simulink model "RLTunningTV"  (R2019b)
settings: Solver=odeN  StartTime=0.0  StopTime=15  FixedStep=0.001  RelTol=1e-3
PreLoadFcn:
  | Vehicle_parameters;
  | hcc_init;
InitFcn:
  | Vehicle_parameters;
  | hcc_init;
values from neighbouring files (symbols this model uses):
  c = (1.596+1.610)/2    (= 1.603)    [Vehicle_parameters.m]
  g = 9.8    [Vehicle_parameters.m]
  gamma = 0.006    [hcc_init.m]
  Jzz = 2050    [Vehicle_parameters.m]
  kx1 = 0.05890269    [hcc_init.m]
  ky1 = 0.04086363    [hcc_init.m]
  kz1 = 0.27516026    [hcc_init.m]
  lf = 1.3265    [Vehicle_parameters.m]
  lr = 1.3685    [Vehicle_parameters.m]
  M = 1360    [Vehicle_parameters.m]
  n = 6    [hcc_init.m]    (also in smoothing_t0.m = 16)
  pbk_gain = 1.0    (= 1)    [hcc_init.m]
  Q_gain = 50.0    (= 50)    [hcc_init.m]
  Qf = [0.0, 0.0 ... (first row only)    [hcc_init.m]
  Qr = [0.0, 0.0 ... (first row only)    [hcc_init.m]
  Reff = 0.323    [Vehicle_parameters.m]
  swa_gain = 45.0    (= 45)    [hcc_init.m]
  umax_m = 4000.0    (= 4000)    [hcc_init.m]
  umin_br = umin_m + umin_b    (= -4500)    [hcc_init.m]
  v = 80    [Vehicle_parameters.m]
  wFx = 0.4    [hcc_init.m]
  wFy = 0.02    [hcc_init.m]
  wGz = 1500.89459504    [hcc_init.m]
undefined symbols (not defined in the file or in its folder): DiscIntNeverNeededParam, LMUX, LMUY, sigbuilder_block
libraries: simulink x10, rllib x1
(part 2 of 3)

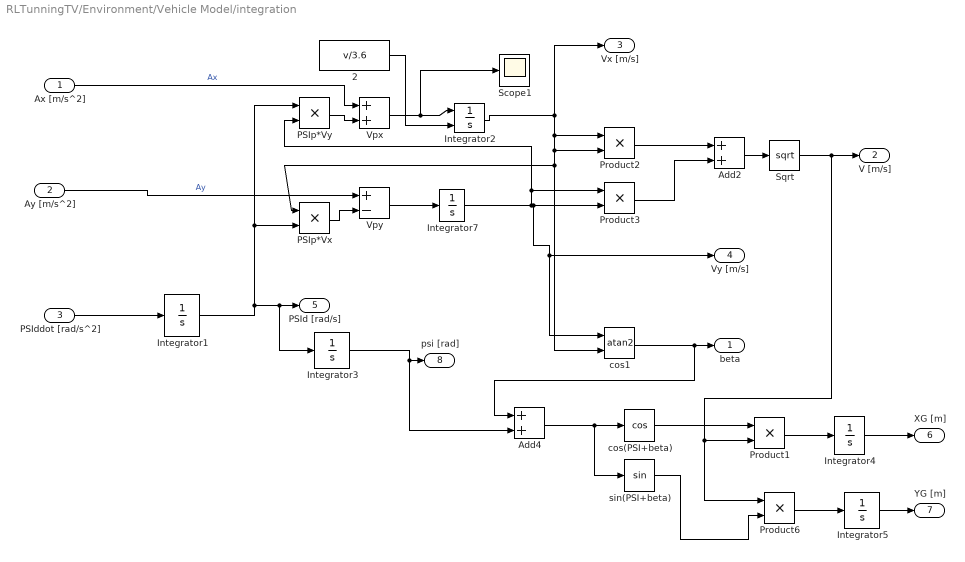
== system RLTunningTV/Environment/Vehicle Model/integration ==
  Ax [m/s^2] : Inport
  Ay [m/s^2] : Inport  Port=2
  PSIddot [rad/s^2] : Inport  Port=3
  2 : Constant  Value=v/3.6
  Add2 : Sum
  Add4 : Sum
  Integrator{1,3..5,7} (5 alike) : Integrator
  Integrator2 : Integrator  InitialConditionSource=external  InitialCondition=v/3.6
  PSIp*Vx : Product  RndMeth=Zero
  PSIp*Vy : Product  RndMeth=Zero
  Product{1..3,6} (4 alike) : Product  RndMeth=Zero
  Scope1 : Scope
  Sqrt : Sqrt  SaturateOnIntegerOverflow=on
  Vpx : Sum
  Vpy : Sum  Inputs=+-
  cos(PSI+beta) : Trigonometry  Operator=cos
  cos1 : Trigonometry  Operator=atan2
  sin(PSI+beta) : Trigonometry
  beta : Outport  VectorParamsAs1DForOutWhenUnconnected=off
  V [m/s] : Outport  Port=2  VectorParamsAs1DForOutWhenUnconnected=off
  Vx [m/s] : Outport  Port=3  VectorParamsAs1DForOutWhenUnconnected=off
  Vy [m/s] : Outport  Port=4  VectorParamsAs1DForOutWhenUnconnected=off
  PSId [rad/s] : Outport  Port=5  VectorParamsAs1DForOutWhenUnconnected=off
  XG [m] : Outport  Port=6  VectorParamsAs1DForOutWhenUnconnected=off
  YG [m] : Outport  Port=7  VectorParamsAs1DForOutWhenUnconnected=off
  psi [rad] : Outport  Port=8  VectorParamsAs1DForOutWhenUnconnected=off
  wires:
  Vpx/1 -> Integrator2/1, Scope1/1
  Integrator5/1 -> YG [m]/1
  Integrator4/1 -> XG [m]/1
  Product1/1 -> Integrator4/1
  Product6/1 -> Integrator5/1
  Add4/1 -> sin(PSI+beta)/1, cos(PSI+beta)/1
  sin(PSI+beta)/1 -> Product6/2
  cos(PSI+beta)/1 -> Product1/1
  Integrator3/1 -> psi [rad]/1, Add4/2
  Sqrt/1 -> Product6/1, Product1/2, V [m/s]/1
  Add2/1 -> Sqrt/1
  Product3/1 -> Add2/2
  Product2/1 -> Add2/1
  cos1/1 -> Add4/1, beta/1
  Ay [m/s^2]/1 -> Vpy/1  "Ay"
  Integrator7/1 -> Product3/2, cos1/1, Vy [m/s]/1, PSIp*Vy/2, Product3/1
  Vpy/1 -> Integrator7/1
  PSIp*Vx/1 -> Vpy/2
  PSIp*Vy/1 -> Vpx/2
  Ax [m/s^2]/1 -> Vpx/1  "Ax"
  Integrator2/1 -> Vx [m/s]/1, PSIp*Vx/1, cos1/2, Product2/2, Product2/1
  PSIddot [rad/s^2]/1 -> Integrator1/1
  Integrator1/1 -> PSIp*Vx/2, PSIp*Vy/1, PSId [rad/s]/1, Integrator3/1
  2/1 -> Integrator2/2

== system RLTunningTV/Environment/Vehicle Model/lateral slip ==
  steering : Inport
  vx : Inport  Port=2
  vy : Inport  Port=3
  psid : Inport  Port=4
  Mux : Mux
  Scope : Scope
  alpha_FL : Subsystem  TreatAsAtomicUnit=on
  alpha_FR : Subsystem  TreatAsAtomicUnit=on
  alpha_RL : Subsystem  TreatAsAtomicUnit=on
  alpha_RR : Subsystem  TreatAsAtomicUnit=on
  alpha[4x1] : Outport  VectorParamsAs1DForOutWhenUnconnected=off
  wires:
  alpha_RL/1(alpha_RL) -> Mux/4
  alpha_RR/1(alpha_RR) -> Mux/3
  alpha_FL/1(alpha_FL) -> Mux/2
  alpha_FR/1(alpha_FR) -> Mux/1, Scope/1
  Mux/1 -> alpha[4x1]/1
  psid/1 -> alpha_FR/4(psid), alpha_FL/4(psid), alpha_RR/3(psid), alpha_RL/3(psid)
  vy/1 -> alpha_FR/3(vy), alpha_FL/3(vy), alpha_RR/2(vy), alpha_RL/2(vy)
  vx/1 -> alpha_FR/2(vx), alpha_FL/2(vx), alpha_RR/1(vx), alpha_RL/1(vx)
  steering/1 -> alpha_FR/1(steering), alpha_FL/1(steering)

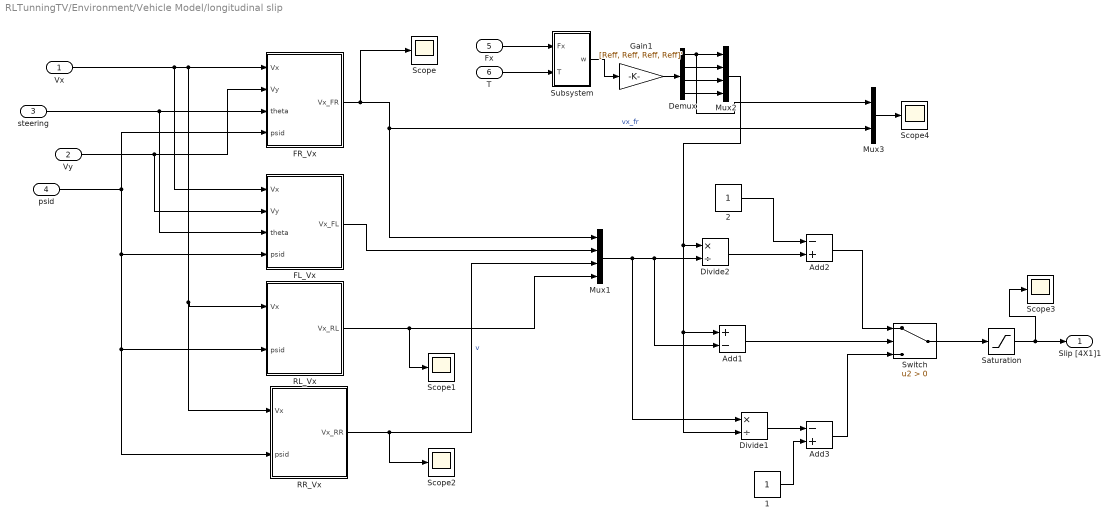
== system RLTunningTV/Environment/Vehicle Model/longitudinal slip ==
  Vx : Inport
  Vy : Inport  Port=2
  steering : Inport  Port=3
  psid : Inport  Port=4
  Fx : Inport  Port=5
  T : Inport  Port=6
  1 : Constant
  2 : Constant
  Add1 : Sum  Inputs=+-
  Add2 : Sum  Inputs=-+
  Add3 : Sum  Inputs=-+
  Demux : Demux
  Divide1 : Product  Inputs=*/
  Divide2 : Product  Inputs=*/
  FL_Vx : Subsystem  TreatAsAtomicUnit=on
  FR_Vx : Subsystem  TreatAsAtomicUnit=on
  Gain1 : Gain  Gain=[Reff, Reff, Reff, Reff]'
  Mux1 : Mux
  Mux2 : Mux
  Mux3 : Mux  Inputs=2
  RL_Vx : Subsystem  TreatAsAtomicUnit=on
  RR_Vx : Subsystem  TreatAsAtomicUnit=on
  Saturation : Saturate  UpperLimit=1  LowerLimit=-1
  Scope{,1..4} (5 alike) : Scope
  Subsystem : Subsystem
  Switch : Switch  Criteria=u2 > Threshold
  Slip [4X1]1 : Outport  VectorParamsAs1DForOutWhenUnconnected=off
  wires:
  T/1 -> Subsystem/2(T)
  Fx/1 -> Subsystem/1(Fx)
  Gain1/1 -> Demux/1
  Add2/1 -> Switch/1
  Add3/1 -> Switch/3
  1/1 -> Add3/2
  Divide1/1 -> Add3/1
  Add1/1 -> Switch/2
  Mux1/1 -> Divide2/2, Add1/2, Divide1/1
  RL_Vx/1(Vx_RL) -> Mux1/4, Scope1/1
  RR_Vx/1(Vx_RR) -> Mux1/3, Scope2/1  "v"
  FL_Vx/1(Vx_FL) -> Mux1/2
  FR_Vx/1(Vx_FR) -> Mux3/2, Mux1/1, Scope/1  "vx_fr"
  2/1 -> Add2/1
  Divide2/1 -> Add2/2
  steering/1 -> FR_Vx/3(theta), FL_Vx/3(theta)
  Vy/1 -> FR_Vx/2(Vy), FL_Vx/2(Vy)
  Subsystem/1(w) -> Gain1/1
  psid/1 -> FR_Vx/4(psid), RL_Vx/2(psid), RR_Vx/2(psid), FL_Vx/4(psid)
  Vx/1 -> RL_Vx/1(Vx), RR_Vx/1(Vx), FR_Vx/1(Vx), FL_Vx/1(Vx)
  Saturation/1 -> Scope3/1, Slip [4X1]1/1
  Demux/1 -> Mux3/1, Mux2/1
  Demux/2 -> Mux2/2
  Demux/3 -> Mux2/3
  Demux/4 -> Mux2/4
  Mux2/1 -> Divide1/2, Add1/1, Divide2/1
  Mux3/1 -> Scope4/1
  Switch/1 -> Saturation/1

== system RLTunningTV/Environment/DCIM/lateral slip/alpha_FL ==
  steering : Inport
  vx : Inport  Port=2
  vy : Inport  Port=3
  psid : Inport  Port=4
  Add : Sum  Inputs=+-
  Add1 : Sum  Inputs=-+
  Add2 : Sum
  Add3 : Sum
  Divide : Product  Inputs=*/
  Gain1 : Gain  Gain=lf
  Product{,1..3} (4 alike) : Product  RndMeth=Zero
  Trigonometric Function2 : Trigonometry  Operator=atan
  cos theta : Trigonometry  Operator=cos
  psid*c : Gain  Gain=c
  sin theta : Trigonometry
  alpha_FL : Outport  VectorParamsAs1DForOutWhenUnconnected=off
  wires:
  vx/1 -> Add/1
  psid/1 -> Gain1/1, psid*c/1
  psid*c/1 -> Add/2
  Add/1 -> Product1/1, Product/1
  steering/1 -> sin theta/1, cos theta/1
  sin theta/1 -> Product2/1, Product/2
  cos theta/1 -> Product3/1, Product1/2
  Product/1 -> Add1/1
  Product1/1 -> Add2/1
  Gain1/1 -> Add3/1
  vy/1 -> Add3/2
  Add3/1 -> Product2/2, Product3/2
  Product2/1 -> Add2/2
  Product3/1 -> Add1/2
  Add1/1 -> Divide/1
  Add2/1 -> Divide/2
  Divide/1 -> Trigonometric Function2/1
  Trigonometric Function2/1 -> alpha_FL/1

== system RLTunningTV/Environment/DCIM/lateral slip/alpha_FR ==
  steering : Inport
  vx : Inport  Port=2
  vy : Inport  Port=3
  psid : Inport  Port=4
  Add : Sum
  Add1 : Sum  Inputs=-+
  Add2 : Sum
  Add3 : Sum
  Divide : Product  Inputs=*/
  Gain : Gain  Gain=c
  Gain1 : Gain  Gain=lf
  Product{,1..3} (4 alike) : Product  RndMeth=Zero
  Trigonometric Function : Trigonometry
  Trigonometric Function1 : Trigonometry  Operator=cos
  Trigonometric Function2 : Trigonometry  Operator=atan
  alpha_FR : Outport  VectorParamsAs1DForOutWhenUnconnected=off
  wires:
  vx/1 -> Add/1
  psid/1 -> Gain1/1, Gain/1
  Gain/1 -> Add/2
  Add/1 -> Product1/1, Product/1
  steering/1 -> Trigonometric Function/1, Trigonometric Function1/1
  Trigonometric Function/1 -> Product2/1, Product/2
  Trigonometric Function1/1 -> Product3/1, Product1/2
  Product/1 -> Add1/1
  Product1/1 -> Add2/1
  Gain1/1 -> Add3/1
  vy/1 -> Add3/2
  Add3/1 -> Product2/2, Product3/2
  Product2/1 -> Add2/2
  Product3/1 -> Add1/2
  Add1/1 -> Divide/1
  Add2/1 -> Divide/2
  Divide/1 -> Trigonometric Function2/1
  Trigonometric Function2/1 -> alpha_FR/1

== system RLTunningTV/Environment/DCIM/lateral slip/alpha_RL ==
  vx : Inport
  vy : Inport  Port=2
  psid : Inport  Port=3
  Add : Sum  Inputs=+-
  Add3 : Sum  Inputs=-+
  Divide : Product  Inputs=*/
  Gain : Gain  Gain=c
  Gain1 : Gain  Gain=lr
  Trigonometric Function2 : Trigonometry  Operator=atan
  alpha_RL : Outport  VectorParamsAs1DForOutWhenUnconnected=off
  wires:
  vx/1 -> Add/1
  psid/1 -> Gain1/1, Gain/1
  Gain/1 -> Add/2
  Add/1 -> Divide/2
  Gain1/1 -> Add3/1
  vy/1 -> Add3/2
  Add3/1 -> Divide/1
  Divide/1 -> Trigonometric Function2/1
  Trigonometric Function2/1 -> alpha_RL/1

== system RLTunningTV/Environment/DCIM/lateral slip/alpha_RR ==
  vx : Inport
  vy : Inport  Port=2
  psid : Inport  Port=3
  Add : Sum
  Add3 : Sum  Inputs=-+
  Divide : Product  Inputs=*/
  Gain : Gain  Gain=c
  Gain1 : Gain  Gain=lr
  Trigonometric Function2 : Trigonometry  Operator=atan
  alpha_RR : Outport  VectorParamsAs1DForOutWhenUnconnected=off
  wires:
  vx/1 -> Add/1
  psid/1 -> Gain1/1, Gain/1
  Gain/1 -> Add/2
  Add/1 -> Divide/2
  Gain1/1 -> Add3/1
  vy/1 -> Add3/2
  Add3/1 -> Divide/1
  Divide/1 -> Trigonometric Function2/1
  Trigonometric Function2/1 -> alpha_RR/1

== system RLTunningTV/Environment/DCIM/longitudinal slip/FL_Vx ==
  Vx : Inport
  Vy : Inport  Port=2
  theta : Inport  Port=3
  psid : Inport  Port=4
  (Vx+PSIp*lf)*sin(theta) : Product  RndMeth=Zero
  (Vx+PSIp*lf)*sin(theta)1 : Product  RndMeth=Zero
  Vx+PSId*lf : Sum
  Vx+PSId*lf1 : Sum  Inputs=+-
  Vx1 : Sum
  cos delta : Trigonometry  Operator=cos
  psip ca/1 : Gain  Gain=c
  psip ca/2 : Gain  Gain=lf
  sin delta : Trigonometry
  Vx_FL : Outport  VectorParamsAs1DForOutWhenUnconnected=off
  wires:
  Vy/1 -> Vx+PSId*lf/1
  psid/1 -> psip ca/1/1, psip ca/2/1
  psip ca/2/1 -> Vx+PSId*lf/2
  Vx+PSId*lf/1 -> (Vx+PSIp*lf)*sin(theta)/1
  theta/1 -> cos delta/1, sin delta/1
  sin delta/1 -> (Vx+PSIp*lf)*sin(theta)/2
  Vx1/1 -> Vx_FL/1
  (Vx+PSIp*lf)*sin(theta)/1 -> Vx1/1
  cos delta/1 -> (Vx+PSIp*lf)*sin(theta)1/1
  Vx/1 -> Vx+PSId*lf1/1
  psip ca/1/1 -> Vx+PSId*lf1/2
  Vx+PSId*lf1/1 -> (Vx+PSIp*lf)*sin(theta)1/2
  (Vx+PSIp*lf)*sin(theta)1/1 -> Vx1/2

== system RLTunningTV/Environment/DCIM/longitudinal slip/FR_Vx ==
  Vx : Inport
  Vy : Inport  Port=2
  theta : Inport  Port=3
  psid : Inport  Port=4
  (Vx+PSIp*lf)*sin(theta)1 : Product  RndMeth=Zero
  (Vy+PSIp*lf)*sin(theta) : Product  RndMeth=Zero
  Vx+PSId*lf : Sum
  Vx+PSId*lf1 : Sum
  Vx2 : Sum
  cos delta : Trigonometry  Operator=cos
  psip ca/1 : Gain  Gain=c
  psip ca/3 : Gain  Gain=lf
  sin delta : Trigonometry
  Vx_FR : Outport  VectorParamsAs1DForOutWhenUnconnected=off
  wires:
  psip ca/3/1 -> Vx+PSId*lf/1
  psid/1 -> psip ca/1/1, psip ca/3/1
  Vx+PSId*lf/1 -> (Vy+PSIp*lf)*sin(theta)/1
  theta/1 -> sin delta/1, cos delta/1
  sin delta/1 -> (Vy+PSIp*lf)*sin(theta)/2
  Vx2/1 -> Vx_FR/1
  (Vy+PSIp*lf)*sin(theta)/1 -> Vx2/1
  cos delta/1 -> (Vx+PSIp*lf)*sin(theta)1/1
  psip ca/1/1 -> Vx+PSId*lf1/2
  Vx+PSId*lf1/1 -> (Vx+PSIp*lf)*sin(theta)1/2
  (Vx+PSIp*lf)*sin(theta)1/1 -> Vx2/2
  Vy/1 -> Vx+PSId*lf/2
  Vx/1 -> Vx+PSId*lf1/1

== system RLTunningTV/Environment/DCIM/longitudinal slip/RL_Vx ==
  Vx : Inport
  psid : Inport  Port=2
  Vx-PSId*c : Sum  Inputs=+-
  psip c : Gain  Gain=c
  Vx_RL : Outport  VectorParamsAs1DForOutWhenUnconnected=off
  wires:
  psid/1 -> psip c/1
  Vx-PSId*c/1 -> Vx_RL/1
  Vx/1 -> Vx-PSId*c/1
  psip c/1 -> Vx-PSId*c/2

== system RLTunningTV/Environment/DCIM/longitudinal slip/RR_Vx ==
  Vx : Inport
  psid : Inport  Port=2
  Vx+PSId*c : Sum
  psip c : Gain  Gain=c
  Vx_RR : Outport  VectorParamsAs1DForOutWhenUnconnected=off
  wires:
  psid/1 -> psip c/1
  Vx+PSId*c/1 -> Vx_RR/1
  Vx/1 -> Vx+PSId*c/1
  psip c/1 -> Vx+PSId*c/2

== system RLTunningTV/Environment/DCIM/longitudinal slip/Subsystem ==
  Fx : Inport
  T : Inport  Port=2
  1/J : Gain  Gain=1./[1.04, 1.04, 1.04 ,1.04]'
  2 : Constant  Value=v/3.6*1/Reff
  Add : Sum  Inputs=-+
  Demux : Demux
  Discrete-Time Integrator{,1..3} (4 alike) : DiscreteIntegrator  InitialConditionSource=external  InitialCondition=v/3.6*1/Reff  SampleTime=0.001  ICPrevOutput=DiscIntNeverNeededParam  ICPrevScaledInput=DiscIntNeverNeededParam
  Mux : Mux
  Reff : Gain  Gain=[Reff, Reff, Reff, Reff]'
  Saturation : Saturate  UpperLimit=inf  LowerLimit=0
  Scope : Scope
  Scope1 : Scope
  w : Outport  VectorParamsAs1DForOutWhenUnconnected=off
  wires:
  Add/1 -> 1/J/1
  Reff/1 -> Add/1
  Saturation/1 -> w/1
  Fx/1 -> Reff/1
  T/1 -> Add/2
  1/J/1 -> Demux/1, Scope/1  "omegap"
  Demux/3 -> Discrete-Time Integrator2/1
  Demux/2 -> Discrete-Time Integrator1/1
  Demux/4 -> Discrete-Time Integrator3/1
  Demux/1 -> Discrete-Time Integrator/1
  Discrete-Time Integrator2/1 -> Mux/3  "omega"
  Discrete-Time Integrator1/1 -> Mux/2
  Discrete-Time Integrator3/1 -> Mux/4
  Discrete-Time Integrator/1 -> Mux/1
  Mux/1 -> Saturation/1, Scope1/1
  2/1 -> Discrete-Time Integrator3/2, Discrete-Time Integrator2/2, Discrete-Time Integrator1/2, Discrete-Time Integrator/2

== system RLTunningTV/Environment/Vehicle Model/lateral slip/alpha_FL ==
  steering : Inport
  vx : Inport  Port=2
  vy : Inport  Port=3
  psid : Inport  Port=4
  Add : Sum  Inputs=+-
  Add1 : Sum  Inputs=-+
  Add2 : Sum
  Add3 : Sum
  Divide : Product  Inputs=*/
  Gain1 : Gain  Gain=lf
  Product{,1..3} (4 alike) : Product  RndMeth=Zero
  Trigonometric Function2 : Trigonometry  Operator=atan
  cos theta : Trigonometry  Operator=cos
  psid*c : Gain  Gain=c
  sin theta : Trigonometry
  alpha_FL : Outport  VectorParamsAs1DForOutWhenUnconnected=off
  wires:
  Trigonometric Function2/1 -> alpha_FL/1
  Divide/1 -> Trigonometric Function2/1
  Add2/1 -> Divide/2
  Add1/1 -> Divide/1
  Product3/1 -> Add1/2
  Product2/1 -> Add2/2
  Add3/1 -> Product3/2, Product2/2
  vy/1 -> Add3/2
  Gain1/1 -> Add3/1
  Product1/1 -> Add2/1
  Product/1 -> Add1/1
  cos theta/1 -> Product1/2, Product3/1
  sin theta/1 -> Product/2, Product2/1
  steering/1 -> cos theta/1, sin theta/1
  Add/1 -> Product/1, Product1/1
  psid*c/1 -> Add/2
  psid/1 -> psid*c/1, Gain1/1
  vx/1 -> Add/1

== system RLTunningTV/Environment/Vehicle Model/lateral slip/alpha_FR ==
  steering : Inport
  vx : Inport  Port=2
  vy : Inport  Port=3
  psid : Inport  Port=4
  Add : Sum
  Add1 : Sum  Inputs=-+
  Add2 : Sum
  Add3 : Sum
  Divide : Product  Inputs=*/
  Gain : Gain  Gain=c
  Gain1 : Gain  Gain=lf
  Product{,1..3} (4 alike) : Product  RndMeth=Zero
  Trigonometric Function : Trigonometry
  Trigonometric Function1 : Trigonometry  Operator=cos
  Trigonometric Function2 : Trigonometry  Operator=atan
  alpha_FR : Outport  VectorParamsAs1DForOutWhenUnconnected=off
  wires:
  Trigonometric Function2/1 -> alpha_FR/1
  Divide/1 -> Trigonometric Function2/1
  Add2/1 -> Divide/2
  Add1/1 -> Divide/1
  Product3/1 -> Add1/2
  Product2/1 -> Add2/2
  Add3/1 -> Product3/2, Product2/2
  vy/1 -> Add3/2
  Gain1/1 -> Add3/1
  Product1/1 -> Add2/1
  Product/1 -> Add1/1
  Trigonometric Function1/1 -> Product1/2, Product3/1
  Trigonometric Function/1 -> Product/2, Product2/1
  steering/1 -> Trigonometric Function1/1, Trigonometric Function/1
  Add/1 -> Product/1, Product1/1
  Gain/1 -> Add/2
  psid/1 -> Gain/1, Gain1/1
  vx/1 -> Add/1

== system RLTunningTV/Environment/Vehicle Model/lateral slip/alpha_RL ==
  vx : Inport
  vy : Inport  Port=2
  psid : Inport  Port=3
  Add : Sum  Inputs=+-
  Add3 : Sum  Inputs=-+
  Divide : Product  Inputs=*/
  Gain : Gain  Gain=c
  Gain1 : Gain  Gain=lr
  Trigonometric Function2 : Trigonometry  Operator=atan
  alpha_RL : Outport  VectorParamsAs1DForOutWhenUnconnected=off
  wires:
  Trigonometric Function2/1 -> alpha_RL/1
  Divide/1 -> Trigonometric Function2/1
  Add3/1 -> Divide/1
  vy/1 -> Add3/2
  Gain1/1 -> Add3/1
  Add/1 -> Divide/2
  Gain/1 -> Add/2
  psid/1 -> Gain/1, Gain1/1
  vx/1 -> Add/1

== system RLTunningTV/Environment/Vehicle Model/lateral slip/alpha_RR ==
  vx : Inport
  vy : Inport  Port=2
  psid : Inport  Port=3
  Add : Sum
  Add3 : Sum  Inputs=-+
  Divide : Product  Inputs=*/
  Gain : Gain  Gain=c
  Gain1 : Gain  Gain=lr
  Trigonometric Function2 : Trigonometry  Operator=atan
  alpha_RR : Outport  VectorParamsAs1DForOutWhenUnconnected=off
  wires:
  Trigonometric Function2/1 -> alpha_RR/1
  Divide/1 -> Trigonometric Function2/1
  Add3/1 -> Divide/1
  vy/1 -> Add3/2
  Gain1/1 -> Add3/1
  Add/1 -> Divide/2
  Gain/1 -> Add/2
  psid/1 -> Gain/1, Gain1/1
  vx/1 -> Add/1

== system RLTunningTV/Environment/Vehicle Model/longitudinal slip/FL_Vx ==
  Vx : Inport
  Vy : Inport  Port=2
  theta : Inport  Port=3
  psid : Inport  Port=4
  (Vx+PSIp*lf)*sin(theta) : Product  RndMeth=Zero
  (Vx+PSIp*lf)*sin(theta)1 : Product  RndMeth=Zero
  Vx+PSId*lf : Sum
  Vx+PSId*lf1 : Sum  Inputs=+-
  Vx1 : Sum
  cos delta : Trigonometry  Operator=cos
  psip ca/1 : Gain  Gain=c
  psip ca/2 : Gain  Gain=lf
  sin delta : Trigonometry
  Vx_FL : Outport  VectorParamsAs1DForOutWhenUnconnected=off
  wires:
  (Vx+PSIp*lf)*sin(theta)1/1 -> Vx1/2
  Vx+PSId*lf1/1 -> (Vx+PSIp*lf)*sin(theta)1/2
  psip ca/1/1 -> Vx+PSId*lf1/2
  Vx/1 -> Vx+PSId*lf1/1
  cos delta/1 -> (Vx+PSIp*lf)*sin(theta)1/1
  (Vx+PSIp*lf)*sin(theta)/1 -> Vx1/1
  Vx1/1 -> Vx_FL/1
  sin delta/1 -> (Vx+PSIp*lf)*sin(theta)/2
  theta/1 -> sin delta/1, cos delta/1
  Vx+PSId*lf/1 -> (Vx+PSIp*lf)*sin(theta)/1
  psip ca/2/1 -> Vx+PSId*lf/2
  psid/1 -> psip ca/2/1, psip ca/1/1
  Vy/1 -> Vx+PSId*lf/1

== system RLTunningTV/Environment/Vehicle Model/longitudinal slip/FR_Vx ==
  Vx : Inport
  Vy : Inport  Port=2
  theta : Inport  Port=3
  psid : Inport  Port=4
  (Vx+PSIp*lf)*sin(theta)1 : Product  RndMeth=Zero
  (Vy+PSIp*lf)*sin(theta) : Product  RndMeth=Zero
  Vx+PSId*lf : Sum
  Vx+PSId*lf1 : Sum
  Vx2 : Sum
  cos delta : Trigonometry  Operator=cos
  psip ca/1 : Gain  Gain=c
  psip ca/3 : Gain  Gain=lf
  sin delta : Trigonometry
  Vx_FR : Outport  VectorParamsAs1DForOutWhenUnconnected=off
  wires:
  Vx/1 -> Vx+PSId*lf1/1
  Vy/1 -> Vx+PSId*lf/2
  (Vx+PSIp*lf)*sin(theta)1/1 -> Vx2/2
  Vx+PSId*lf1/1 -> (Vx+PSIp*lf)*sin(theta)1/2
  psip ca/1/1 -> Vx+PSId*lf1/2
  cos delta/1 -> (Vx+PSIp*lf)*sin(theta)1/1
  (Vy+PSIp*lf)*sin(theta)/1 -> Vx2/1
  Vx2/1 -> Vx_FR/1
  sin delta/1 -> (Vy+PSIp*lf)*sin(theta)/2
  theta/1 -> cos delta/1, sin delta/1
  Vx+PSId*lf/1 -> (Vy+PSIp*lf)*sin(theta)/1
  psid/1 -> psip ca/3/1, psip ca/1/1
  psip ca/3/1 -> Vx+PSId*lf/1

== system RLTunningTV/Environment/Vehicle Model/longitudinal slip/RL_Vx ==
  Vx : Inport
  psid : Inport  Port=2
  Vx-PSId*c : Sum  Inputs=+-
  psip c : Gain  Gain=c
  Vx_RL : Outport  VectorParamsAs1DForOutWhenUnconnected=off
  wires:
  psip c/1 -> Vx-PSId*c/2
  Vx/1 -> Vx-PSId*c/1
  Vx-PSId*c/1 -> Vx_RL/1
  psid/1 -> psip c/1

== system RLTunningTV/Environment/Vehicle Model/longitudinal slip/RR_Vx ==
  Vx : Inport
  psid : Inport  Port=2
  Vx+PSId*c : Sum
  psip c : Gain  Gain=c
  Vx_RR : Outport  VectorParamsAs1DForOutWhenUnconnected=off
  wires:
  psip c/1 -> Vx+PSId*c/2
  Vx/1 -> Vx+PSId*c/1
  Vx+PSId*c/1 -> Vx_RR/1
  psid/1 -> psip c/1

== system RLTunningTV/Environment/Vehicle Model/longitudinal slip/Subsystem ==
  Fx : Inport
  T : Inport  Port=2
  1/J : Gain  Gain=1./[1.04, 1.04, 1.04 ,1.04]'
  2 : Constant  Value=v/3.6*1/Reff
  Add : Sum  Inputs=-+
  Demux : Demux
  Discrete-Time Integrator{,1..3} (4 alike) : DiscreteIntegrator  InitialConditionSource=external  InitialCondition=v/3.6*1/Reff  SampleTime=0.001  ICPrevOutput=DiscIntNeverNeededParam  ICPrevScaledInput=DiscIntNeverNeededParam
  Mux : Mux
  Reff : Gain  Gain=[Reff, Reff, Reff, Reff]'
  Saturation : Saturate  UpperLimit=inf  LowerLimit=0
  Scope : Scope
  Scope1 : Scope
  w : Outport  VectorParamsAs1DForOutWhenUnconnected=off
  wires:
  Mux/1 -> Scope1/1, Saturation/1
  Discrete-Time Integrator/1 -> Mux/1
  Discrete-Time Integrator3/1 -> Mux/4
  Discrete-Time Integrator1/1 -> Mux/2
  Discrete-Time Integrator2/1 -> Mux/3  "omega"
  Demux/1 -> Discrete-Time Integrator/1
  Demux/4 -> Discrete-Time Integrator3/1
  Demux/2 -> Discrete-Time Integrator1/1
  Demux/3 -> Discrete-Time Integrator2/1
  1/J/1 -> Scope/1, Demux/1  "omegap"
  T/1 -> Add/2
  Fx/1 -> Reff/1
  Saturation/1 -> w/1
  Reff/1 -> Add/1
  Add/1 -> 1/J/1
  2/1 -> Discrete-Time Integrator3/2, Discrete-Time Integrator2/2, Discrete-Time Integrator1/2, Discrete-Time Integrator/2

== matlab function RLTunningTV/Environment/Embedded MATLAB Function ==
  data: wFx input; wFy input; wFz input; wFx1 output; kx1 input; ky1 input; kz1 input; SWA input; dSWA input; Q input; Vx input; wFy1 output; wFz1 output
function [wFx1, wFy1, wFz1] = fcn(wFx,wFy,wFz,kx1,ky1,kz1,SWA,dSWA,Q,Vx)
% This block supports the Embedded MATLAB subset.
% See the help menu for details.

Qnom = 8000.0;
Vxnom = 100.0/3.6;

wx1 = wFx*(1+kx1*abs(Q)/Qnom);
wy1 = wFy*(1+ky1*(Vx/Vxnom)*(Vx/Vxnom)*abs(SWA)/(2*pi));
wz1 = wFz*(1+kz1*abs(dSWA)/(2*pi));


% wx1 = wFx + kx1*abs(Q)/Qnom;
% wy1 = wFy + ky1*(Vx/Vxnom)*(Vx/Vxnom)*abs(SWA)/(2*pi);
% wz1 = wFz + kz1*abs(dSWA)/(2*pi);


wFx1 = wx1*(1+sign(wx1))/2.0;
wFy1 = wy1*(1+sign(wy1))/2.0;
wFz1 = wz1*(1+sign(wz1))/2.0;

== matlab function RLTunningTV/Environment/DCIM/Tire_model/Pacejka_Fx ==
  data: slip_FR input; slip_FL input; slip_RR input; slip_RL input; Fx output; Fz_FR input; Fz_FL input; Fz_RR input; Fz_RL input
function Fx   = fcn( slip_FR,  slip_FL,  slip_RR,  slip_RL, Fz_FR, Fz_FL, Fz_RR, Fz_RL)

my_mu=0.5;


%[SCALING_COEFFICIENTS]
LFZO                  	= 1;		% scale factor of nominal (rated) load
LCX                   	= 1;		% scale factor of Fx shape factor
LMUX                  	= 1;	    % scale factor of Fx peak friction coefficient
LEX                   	= 1;		% scale factor of Fx curvature factor
LKX                   	= 1;		% scale factor of Fx slip stiffness
LHX                   	= 1;	    % scale factor of Fx horizontal shfit
LVX                   	= 1;		% scale factor of Fx vertical shift
LGAX			        = 1;		% scale factor of camber for Fx  
LCY                   	= 1;		% scale factor of Fy shape factor
LMUY                  	= 1;		% scale factor of Fy peak friction coefficient
LEY                   	= 1;		% scale factor of Fy curvature factor
LKY                   	= 1;		% scale factor of Fy cornering stiffness
LHY                   	= 1;		% scale factor of Fy horizontal shift
LVY                   	= 1;		% scale factor of Fy vertical shift
LGAY                  	= 1;		% scale factor of camber for Fy
LTR                   	= 1;		% scale factor of peak of pneumatic trail
LRES                  	= 1;		% scale factor for offset of residual torque
LGAZ                  	= 1;		% scale factor of camber for Mz        
LXAL                  	= 1;		% scale factor of alpha infulence on Fx
LYKA                  	= 1;		% scale factor of kappa influence on Fy
LVYKA                 	= 1;		% scale factor of kappa induced Fy
LS                    	= 1;		% scale factor of Mz moment arm of Fx
LSGKP                 	= 1;		% scale factor of relaxation length of Fx
LSGAL                 	= 1;		% scale factor of relaxation length of Fy
LGYR                  	= 1;		% scale factor of gyroscopic torque
LMX                   	= 1;		% scale factor of overturning couple stiffness
LVMX			        = 1;		% scale factor of Mx vertical shift  
LMY                   	= 1;		% scale factor of rolling resistance torque

%[LONGITUDINAL_COEFFICIENTS]
PCX1                  	=  1.6055;	    % shape factor Cfx for longitudinal force 
PDX1                  	=  1.1703;	    % longitudinal friction Mux at FzNom
PDX2                  	= -0.081328;	% variation of friction Mux with load
PDX3			        =  0;	 	    % variation of friction Mux with camber    
PEX1                  	=  0.53409;	    % longitudinal curvature Efx at FzNom
PEX2                  	= -0.019956;	% variation of curvature Efx with load
PEX3                  	=  0.18089;  	% variation of curvature Efx with squared load 
PEX4                  	=  2.9951e-07;	% factor in curvature Efx while driving
PKX1                  	=  36.411;	    % longitudinal slip stiffness Kfx/Fz at FzNom
PKX2                  	=  0.12615;	    % variation of slip stiffness Kfx/Fz with load
PKX3                  	=  0.51289;	    % exponent in slip stiffness Kfx/Fz with load
PHX1                  	=  0;		    % horizontal shift Shx at Fznom
PHX2                  	=  0;		    % variation of shift Shx with load
PVX1                  	=  0;		    % vertical shift Svx/Fz at FzNom
PVX2                  	=  0;		    % variation of shift Svx/Fz with load
RBX1                  	=  18.456;	    % slope factor for combined slip Fx reduction
RBX2                  	=  16.314;	    % variation of slope Fx reduction with Kappa
RCX1                  	=  1.091;	    % shape factor for combined slip Fx reduction
REX1			        =  0;		    % curvature factor of combined Fx     
REX2			        =  0;		    % curvature factor of combined Fx with load   
RHX1                  	=  0.0058715;	% shift factor for combined slip Fx reduction
PTX1                  	=  1.5;		    % relaxation length Sig_Kappa/Fz at FzNom
PTX2                  	=  0.180096;	% variation of Sig_Kappa/Fz with load  
PTX3                  	= -0.15;		% variation of Sig_Kappa/Fz with exponent of load

FNOMIN                	= 6500;		    % nominal wheel load
g = 9.8;
% Pacejka parameters

dfz_FR    =   (Fz_FR - FNOMIN)/FNOMIN ; 
S_hx_FR   =   (PHX1 + PHX2*dfz_FR)*LHX ;
K_x_FR    =    slip_FR + S_hx_FR;                         
     
C_x_FR    =    PCX1*LCX;

% LMUX                  	= my_mu/(PDX1 + PDX2*dfz_FR);
mux_FR    =   (PDX1 + PDX2*dfz_FR)*LMUX;
D_x_FR    =   mux_FR * Fz_FR;
E_x_FR    =   (PEX1 + PEX2*dfz_FR + PEX3*dfz_FR^2)*(1 - PEX4*sign(K_x_FR))*LEX;
K_xk_FR   =    Fz_FR*(PKX1 + PKX2*dfz_FR)*exp(PKX3*dfz_FR);
B_x_FR    =    (K_xk_FR)/(C_x_FR*D_x_FR);
S_Vx_FR        = Fz_FR * (PVX1 + PVX2 * dfz_FR) * LVX * LMUX;

Fx_FR = D_x_FR*sin(C_x_FR*atan(B_x_FR*K_x_FR-E_x_FR*(B_x_FR*K_x_FR-atan(B_x_FR*K_x_FR))))+S_Vx_FR;

% FL

dfz_FL    =   (Fz_FL - FNOMIN)/FNOMIN ; 
S_hx_FL   =   (PHX1 + PHX2*dfz_FL)*LHX ;
K_x_FL    =    slip_FL + S_hx_FL;                         
     
C_x_FL    =    PCX1*LCX;
mux_FL    =   (PDX1 + PDX2*dfz_FL)*LMUX;
D_x_FL    =   mux_FL * Fz_FL;
E_x_FL    =   (PEX1 + PEX2*dfz_FL + PEX3*dfz_FL^2)*(1 - PEX4*sign(K_x_FL))*LEX;
K_xk_FL   =    Fz_FL*(PKX1 + PKX2*dfz_FL)*exp(PKX3*dfz_FL);
B_x_FL    =    (K_xk_FL)/(C_x_FL*D_x_FL);
S_Vx_FL        = Fz_FL * (PVX1 + PVX2 * dfz_FL) * LVX * LMUX;

Fx_FL = D_x_FL*sin(C_x_FL*atan(B_x_FL*K_x_FL-E_x_FL*(B_x_FL*K_x_FL-atan(B_x_FL*K_x_FL))))+S_Vx_FL;

% RR

dfz_RR    =   (Fz_RR - FNOMIN)/FNOMIN ; 
S_hx_RR   =   (PHX1 + PHX2*dfz_RR)*LHX ;
K_x_RR    =    slip_RR + S_hx_RR;                         
     
C_x_RR    =    PCX1*LCX;
mux_RR    =   (PDX1 + PDX2*dfz_RR)*LMUX;
D_x_RR    =    mux_RR *Fz_RR;
E_x_RR    =   (PEX1 + PEX2*dfz_RR + PEX3*dfz_RR^2)*(1 - PEX4*sign(K_x_RR))*LEX;
K_xk_RR   =    Fz_RR*(PKX1 + PKX2*dfz_RR)*exp(PKX3*dfz_RR);
B_x_RR    =    (K_xk_RR)/(C_x_RR*D_x_RR);
S_Vx_RR        = Fz_RR * (PVX1 + PVX2 * dfz_RR) * LVX * LMUX;

Fx_RR = D_x_RR*sin(C_x_RR*atan(B_x_RR*K_x_RR - E_x_RR*(B_x_RR*K_x_RR-atan(B_x_RR*K_x_RR))))+S_Vx_RR;

% RL

dfz_RL    =   (Fz_RL - FNOMIN)/FNOMIN ; 
S_hx_RL   =   (PHX1 + PHX2*dfz_RL)*LHX ;
K_x_RL    =    slip_RL + S_hx_RL;                         
     
C_x_RL    =    PCX1*LCX;
mux_RL    =   (PDX1 + PDX2*dfz_RL)*LMUX;
D_x_RL    =    mux_RL*Fz_RL;
E_x_RL    =   (PEX1 + PEX2*dfz_RL + PEX3*dfz_RL^2)*(1 - PEX4*sign(K_x_RL))*LEX;
K_xk_RL   =    Fz_RL*(PKX1 + PKX2*dfz_RL)*exp(PKX3*dfz_RL);
B_x_RL    =    (K_xk_RL)/(C_x_RL*D_x_RL);
S_Vx_RL        = Fz_RL * (PVX1 + PVX2 * dfz_RL) * LVX * LMUX;

Fx_RL     =    D_x_RL*sin(C_x_RL*atan(B_x_RL*K_x_RL - E_x_RL*(B_x_RL*K_x_RL-atan(B_x_RL*K_x_RL))))+S_Vx_RL;

Fx = [Fx_FR, Fx_FL, Fx_RR, Fx_RL]';
mux = [mux_FR, mux_FL, mux_RR, mux_RL]';

== matlab function RLTunningTV/Environment/Vehicle Model/Tire_model/Pacejka_Fy ==
  data: Fy output; alphaFR input; alphaFL input; alphaRR input; alphaRL input; Fz_FR input; Fz_FL input; Fz_RR input; Fz_RL input; muy output; LMUY input
function [Fy, muy] = fcn(alphaFR , alphaFL, alphaRR, alphaRL,   Fz_FR, Fz_FL, Fz_RR, Fz_RL,LMUY)

m = 1360;             % vehicle mass[kg]
g = 9.8;


%[SCALING_COEFFICIENTS]
LFZO                  	= 1;		% scale factor of nominal (rated) load
LCX                   	= 1;		% scale factor of Fx shape factor
LMUX                  	= 1;	    % scale factor of Fx peak friction coefficient
LEX                   	= 1;		% scale factor of Fx curvature factor
LKX                   	= 1;		% scale factor of Fx slip stiffness
LHX                   	= 1;	    % scale factor of Fx horizontal shfit
LVX                   	= 1;		% scale factor of Fx vertical shift
LGAX			        = 1;		% scale factor of camber for Fx  
LCY                   	= 1;		% scale factor of Fy shape factor
% LMUY                  	= 0.5;		% scale factor of Fy peak friction coefficient
LEY                   	= 1;		% scale factor of Fy curvature factor
LKY                   	= 1;		% scale factor of Fy cornering stiffness
LHY                   	= 1;		% scale factor of Fy horizontal shift
LVY                   	= 1;		% scale factor of Fy vertical shift
LGAY                  	= 1;		% scale factor of camber for Fy
LTR                   	= 1;		% scale factor of peak of pneumatic trail
LRES                  	= 1;		% scale factor for offset of residual torque
LGAZ                  	= 1;		% scale factor of camber for Mz        
LXAL                  	= 1;		% scale factor of alpha infulence on Fx
LYKA                  	= 1;		% scale factor of kappa influence on Fy
LVYKA                 	= 1;		% scale factor of kappa induced Fy
LS                    	= 1;		% scale factor of Mz moment arm of Fx
LSGKP                 	= 1;		% scale factor of relaxation length of Fx
LSGAL                 	= 1;		% scale factor of relaxation length of Fy
LGYR                  	= 1;		% scale factor of gyroscopic torque
LMX                   	= 1;		% scale factor of overturning couple stiffness
LVMX			        = 1;		% scale factor of Mx vertical shift  
LMY                   	= 1;		% scale factor of rolling resistance torque




%[LATERAL_COEFFICIENTS]
PCY1                  	=  2.1322;	          % shape factor Cfy for lateral forces
PDY1                  	=  1.0283;	          % lateral friction Muy at FzNom
PDY2                  	= -0.16758;	          % variation of friction Muy with load
PDY3                  	= -1.5821;	          % variation of friction Muy with squared camber
PEY1                  	=  0.33443;	          % lateral curvature Efy at FzNom
PEY2                  	= -1.8733;	          % variation of curvature Efy with load
PEY3                  	= -0.13136;	          % zero order camber dependency of curvature Efy
PEY4                  	= -11.677;	          % variation of curvature Efy with camber
PKY1                  	= -20.505;	          % maximum value of stiffness Kfy/FzNom
PKY2                  	=  2.0284;	          % load at which Kfy reaches maximum value
PKY3                  	=  0.89994;	          % variation of Kfy/Fznom with camber
PHY1                  	=  0.0031377;	      % horizontal shift Shy at FzNom
PHY2                  	=  0.00051596;	      % variation of shift Shy with load
PHY3                  	=  0.039251;	      % variation of shift Shy with camber
PVY1                  	=  0.026365;	      % vertical shift in Svy/Fz at FzNom
PVY2                  	= -0.0062119;    	  % variation of shift Svy/Fz with load
PVY3                  	= -0.41389;	          % variation of shift Svy/Fz with camber
PVY4                  	= -0.048038;	      % variation of shift Svy/Fz with camber and load
RBY1                  	=  22.003;	          % slope factor for combined Fy reduction
RBY2                  	= -13.623;	          % variation of slope Fy reduction with Alpha
RBY3                  	= -0.0093616;	      % shfit term for alpha in slope Fy reduction
RCY1                  	=  0.98294;	          % shape factor for combined Fy reduction
REY1			        =  0;		          % Curvature factor of combined Fy     
REY2			        =  0;		          % Curvature factor of combined Fy with load   
RHY1                  	= -9.1492e-11;	      % shift factor for combined Fy reduction
RHY2			        =  0;		          % shift factor for combined Fy reduction with load  
RVY1                  	=  22.965;	          % kappa induced side force Svyk/Muy*Fz at FzNom
RVY2                  	=  0.37981;	          % variation of Svyk/Muy*Fz with load 
RVY3                  	=  1.8552;	          % variation of Svyk/Muy*Fz with camber
RVY4                  	=  0.08767;	          % variation of Svyk/Muy*Fz with alpha
RVY5                  	= -8.8234e-11;        % variation of Svyk/Muy*Fz with kappa
RVY6                  	=  0.90374;	          % variation of Svyk/Muy*Fz with atan(kappa)
PTY1                  	=  1.75;		      % peak value of relaxation length Sig_Alpha
PTY2                  	=  1.35;		      % shape factor for Sig_alpha

FNOMIN                	= 6500;		    % nominal wheel load


PHY1_L    = PHY1;
PHY2_L    = PHY2;
PHY1_R    = -PHY1;
PHY2_R    = -PHY2;


PVY1_L    = PVY1;
PVY2_L    = PVY2;
PVY1_R    = -PVY1;
PVY2_R    = -PVY2;

% FR

dfz_FR    =   (Fz_FR - FNOMIN)/FNOMIN ;                    
     
S_H_FR = PHY1_R + PHY2_R*dfz_FR;
alpha_y_FR = alphaFR + S_H_FR;
C_y_FR    =     PCY1 *LCY;
muy_FR    =    (PDY1 + PDY2*dfz_FR)*LMUY;
D_y_FR    =     muy_FR * Fz_FR;
% E_y_FR    =    (PEY1  + PEY2 *dfz_FR + PEY3 *dfz_FR^2)*(1 - PEY4  *sign(alpha_y_FR ))*LEY;
E_y_FR    =    (PEY1  + PEY2 *dfz_FR)*(1 - PEY3  *sign(alpha_y_FR))*LEY;
K_yk_FR   =     PKY1*FNOMIN*sin(PKY2*atan(Fz_FR/(PKY2*FNOMIN)))*LKY ;
B_y_FR    =    (K_yk_FR)/(C_y_FR*D_y_FR);

S_Vy_FR        = Fz_FR * ((PVY1_R+ PVY2_R* dfz_FR) * LVY )* LMUY ;

Fy_FR = D_y_FR*sin(C_y_FR*atan(B_y_FR*alpha_y_FR - E_y_FR*(B_y_FR*alpha_y_FR - atan(B_y_FR*alpha_y_FR))))+S_Vy_FR;

% dfz_ = 1
% FL
% Fz_FL = m*g/2;



dfz_FL    =   (Fz_FL - FNOMIN)/FNOMIN ;                    
     
S_H_FL = PHY1_L + PHY2_L*dfz_FL;
alpha_y_FL = alphaFL + S_H_FL;
C_y_FL    =     PCY1 *LCY;
muy_FL    =    (PDY1 + PDY2*dfz_FL)*LMUY;
D_y_FL    =     muy_FL * Fz_FL;
E_y_FL    =    (PEY1  + PEY2 *dfz_FL)*(1 - PEY3  *sign(alpha_y_FL))*LEY;
K_yk_FL   =     PKY1*FNOMIN*sin(PKY2*atan(Fz_FL/(PKY2*FNOMIN)))*LKY ;
B_y_FL    =    (K_yk_FL)/(C_y_FL*D_y_FL);

S_Vy_FL        = Fz_FL * ((PVY1_L+ PVY2_L* dfz_FL) * LVY )* LMUY ;


Fy_FL = D_y_FL*sin(C_y_FL*atan(B_y_FL*alpha_y_FL - E_y_FL*(B_y_FL*alpha_y_FL - atan(B_y_FL*alpha_y_FL))))+S_Vy_FL;

% RR
% Fz_RR = m*g/2;
dfz_RR    =   (Fz_RR - FNOMIN)/FNOMIN ;                    
     
S_H_RR = PHY1_R + PHY2_R*dfz_RR;
alpha_y_RR = alphaRR + S_H_RR;
C_y_RR    =     PCY1 *LCY;
muy_RR    =    (PDY1 + PDY2*dfz_RR)*LMUY;
D_y_RR    =     muy_RR * Fz_RR;
E_y_RR    =    (PEY1  + PEY2 *dfz_RR)*(1 - PEY3*sign(alpha_y_RR))*LEY;
K_yk_RR   =     PKY1*FNOMIN*sin(PKY2*atan(Fz_RR/(PKY2*FNOMIN)))*LKY ;
B_y_RR    =    (K_yk_RR)/(C_y_RR*D_y_RR);
S_Vy_RR        = Fz_RR * ((PVY1_R+ PVY2_R* dfz_RR) * LVY )* LMUY ;

Fy_RR = D_y_RR*sin(C_y_RR*atan(B_y_RR*alpha_y_RR - E_y_RR*(B_y_RR*alpha_y_RR - atan(B_y_RR*alpha_y_RR))))+S_Vy_RR;

% RL
% Fz_RL = m*g/2;
dfz_RL    =   (Fz_RL - FNOMIN)/FNOMIN ;                    
 
S_H_RL = PHY1_L + PHY2_L*dfz_RL;
alpha_y_RL = alphaRL + S_H_RL;
C_y_RL    =     PCY1 *LCY;
muy_RL    =    (PDY1 + PDY2*dfz_RL)*LMUY;
D_y_RL    =     muy_RL * Fz_RL;
E_y_RL    =    (PEY1  + PEY2 *dfz_RL)*(1 - PEY3  *sign(alpha_y_RL))*LEY;
K_yk_RL   =     PKY1*FNOMIN*sin(PKY2*atan(Fz_RL/(PKY2*FNOMIN)))*LKY ;
B_y_RL    =    (K_yk_RL)/(C_y_RL*D_y_RL);
S_Vy_RL        = Fz_RL * ((PVY1_L+ PVY2_L* dfz_RL) * LVY )* LMUY ;

Fy_RL = D_y_RL*sin(C_y_RL*atan(B_y_RL*alpha_y_RL - E_y_RL*(B_y_RL*alpha_y_RL - atan(B_y_RL*alpha_y_RL))))+S_Vy_RL;

Fy = [Fy_FR, Fy_FL, Fy_RR, Fy_RL]';
muy = [muy_FR, muy_FL, muy_RR, muy_RL]';

== matlab function RLTunningTV/Environment/Vehicle Model/Tire_model/Pacejka_Fx ==
  data: slip_FR input; slip_FL input; slip_RR input; slip_RL input; Fx output; Fz_FR input; Fz_FL input; Fz_RR input; Fz_RL input; mux output; LMUX input
function [Fx, mux]  = fcn( slip_FR,  slip_FL,  slip_RR,  slip_RL, Fz_FR, Fz_FL, Fz_RR, Fz_RL,LMUX)

my_mu=0.5;


%[SCALING_COEFFICIENTS]
LFZO                  	= 1;		% scale factor of nominal (rated) load
LCX                   	= 1;		% scale factor of Fx shape factor
% LMUX                  	= 0.5;	    % scale factor of Fx peak friction coefficient
LEX                   	= 1;		% scale factor of Fx curvature factor
LKX                   	= 1;		% scale factor of Fx slip stiffness
LHX                   	= 1;	    % scale factor of Fx horizontal shfit
LVX                   	= 1;		% scale factor of Fx vertical shift
LGAX			        = 1;		% scale factor of camber for Fx  
LCY                   	= 1;		% scale factor of Fy shape factor
LMUY                  	= 1;		% scale factor of Fy peak friction coefficient
LEY                   	= 1;		% scale factor of Fy curvature factor
LKY                   	= 1;		% scale factor of Fy cornering stiffness
LHY                   	= 1;		% scale factor of Fy horizontal shift
LVY                   	= 1;		% scale factor of Fy vertical shift
LGAY                  	= 1;		% scale factor of camber for Fy
LTR                   	= 1;		% scale factor of peak of pneumatic trail
LRES                  	= 1;		% scale factor for offset of residual torque
LGAZ                  	= 1;		% scale factor of camber for Mz        
LXAL                  	= 1;		% scale factor of alpha infulence on Fx
LYKA                  	= 1;		% scale factor of kappa influence on Fy
LVYKA                 	= 1;		% scale factor of kappa induced Fy
LS                    	= 1;		% scale factor of Mz moment arm of Fx
LSGKP                 	= 1;		% scale factor of relaxation length of Fx
LSGAL                 	= 1;		% scale factor of relaxation length of Fy
LGYR                  	= 1;		% scale factor of gyroscopic torque
LMX                   	= 1;		% scale factor of overturning couple stiffness
LVMX			        = 1;		% scale factor of Mx vertical shift  
LMY                   	= 1;		% scale factor of rolling resistance torque

%[LONGITUDINAL_COEFFICIENTS]
PCX1                  	=  1.6055;	    % shape factor Cfx for longitudinal force 
PDX1                  	=  1.1703;	    % longitudinal friction Mux at FzNom
PDX2                  	= -0.081328;	% variation of friction Mux with load
PDX3			        =  0;	 	    % variation of friction Mux with camber    
PEX1                  	=  0.53409;	    % longitudinal curvature Efx at FzNom
PEX2                  	= -0.019956;	% variation of curvature Efx with load
PEX3                  	=  0.18089;  	% variation of curvature Efx with squared load 
PEX4                  	=  2.9951e-07;	% factor in curvature Efx while driving
PKX1                  	=  36.411;	    % longitudinal slip stiffness Kfx/Fz at FzNom
PKX2                  	=  0.12615;	    % variation of slip stiffness Kfx/Fz with load
PKX3                  	=  0.51289;	    % exponent in slip stiffness Kfx/Fz with load
PHX1                  	=  0;		    % horizontal shift Shx at Fznom
PHX2                  	=  0;		    % variation of shift Shx with load
PVX1                  	=  0;		    % vertical shift Svx/Fz at FzNom
PVX2                  	=  0;		    % variation of shift Svx/Fz with load
RBX1                  	=  18.456;	    % slope factor for combined slip Fx reduction
RBX2                  	=  16.314;	    % variation of slope Fx reduction with Kappa
RCX1                  	=  1.091;	    % shape factor for combined slip Fx reduction
REX1			        =  0;		    % curvature factor of combined Fx     
REX2			        =  0;		    % curvature factor of combined Fx with load   
RHX1                  	=  0.0058715;	% shift factor for combined slip Fx reduction
PTX1                  	=  1.5;		    % relaxation length Sig_Kappa/Fz at FzNom
PTX2                  	=  0.180096;	% variation of Sig_Kappa/Fz with load  
PTX3                  	= -0.15;		% variation of Sig_Kappa/Fz with exponent of load

FNOMIN                	= 6500;		    % nominal wheel load
g = 9.8;
% Pacejka parameters

dfz_FR    =   (Fz_FR - FNOMIN)/FNOMIN ; 
S_hx_FR   =   (PHX1 + PHX2*dfz_FR)*LHX ;
K_x_FR    =    slip_FR + S_hx_FR;                         
     
C_x_FR    =    PCX1*LCX;

% LMUX                  	= my_mu/(PDX1 + PDX2*dfz_FR);
mux_FR    =   (PDX1 + PDX2*dfz_FR)*LMUX;
D_x_FR    =   mux_FR * Fz_FR;
E_x_FR    =   (PEX1 + PEX2*dfz_FR + PEX3*dfz_FR^2)*(1 - PEX4*sign(K_x_FR))*LEX;
K_xk_FR   =    Fz_FR*(PKX1 + PKX2*dfz_FR)*exp(PKX3*dfz_FR);
B_x_FR    =    (K_xk_FR)/(C_x_FR*D_x_FR);
S_Vx_FR        = Fz_FR * (PVX1 + PVX2 * dfz_FR) * LVX * LMUX;

Fx_FR = D_x_FR*sin(C_x_FR*atan(B_x_FR*K_x_FR-E_x_FR*(B_x_FR*K_x_FR-atan(B_x_FR*K_x_FR))))+S_Vx_FR;

% FL

dfz_FL    =   (Fz_FL - FNOMIN)/FNOMIN ; 
S_hx_FL   =   (PHX1 + PHX2*dfz_FL)*LHX ;
K_x_FL    =    slip_FL + S_hx_FL;                         
     
C_x_FL    =    PCX1*LCX;
mux_FL    =   (PDX1 + PDX2*dfz_FL)*LMUX;
D_x_FL    =   mux_FL * Fz_FL;
E_x_FL    =   (PEX1 + PEX2*dfz_FL + PEX3*dfz_FL^2)*(1 - PEX4*sign(K_x_FL))*LEX;
K_xk_FL   =    Fz_FL*(PKX1 + PKX2*dfz_FL)*exp(PKX3*dfz_FL);
B_x_FL    =    (K_xk_FL)/(C_x_FL*D_x_FL);
S_Vx_FL        = Fz_FL * (PVX1 + PVX2 * dfz_FL) * LVX * LMUX;

Fx_FL = D_x_FL*sin(C_x_FL*atan(B_x_FL*K_x_FL-E_x_FL*(B_x_FL*K_x_FL-atan(B_x_FL*K_x_FL))))+S_Vx_FL;

% RR

dfz_RR    =   (Fz_RR - FNOMIN)/FNOMIN ; 
S_hx_RR   =   (PHX1 + PHX2*dfz_RR)*LHX ;
K_x_RR    =    slip_RR + S_hx_RR;                         
     
C_x_RR    =    PCX1*LCX;
mux_RR    =   (PDX1 + PDX2*dfz_RR)*LMUX;
D_x_RR    =    mux_RR *Fz_RR;
E_x_RR    =   (PEX1 + PEX2*dfz_RR + PEX3*dfz_RR^2)*(1 - PEX4*sign(K_x_RR))*LEX;
K_xk_RR   =    Fz_RR*(PKX1 + PKX2*dfz_RR)*exp(PKX3*dfz_RR);
B_x_RR    =    (K_xk_RR)/(C_x_RR*D_x_RR);
S_Vx_RR        = Fz_RR * (PVX1 + PVX2 * dfz_RR) * LVX * LMUX;

Fx_RR = D_x_RR*sin(C_x_RR*atan(B_x_RR*K_x_RR - E_x_RR*(B_x_RR*K_x_RR-atan(B_x_RR*K_x_RR))))+S_Vx_RR;

% RL

dfz_RL    =   (Fz_RL - FNOMIN)/FNOMIN ; 
S_hx_RL   =   (PHX1 + PHX2*dfz_RL)*LHX ;
K_x_RL    =    slip_RL + S_hx_RL;                         
     
C_x_RL    =    PCX1*LCX;
mux_RL    =   (PDX1 + PDX2*dfz_RL)*LMUX;
D_x_RL    =    mux_RL*Fz_RL;
E_x_RL    =   (PEX1 + PEX2*dfz_RL + PEX3*dfz_RL^2)*(1 - PEX4*sign(K_x_RL))*LEX;
K_xk_RL   =    Fz_RL*(PKX1 + PKX2*dfz_RL)*exp(PKX3*dfz_RL);
B_x_RL    =    (K_xk_RL)/(C_x_RL*D_x_RL);
S_Vx_RL        = Fz_RL * (PVX1 + PVX2 * dfz_RL) * LVX * LMUX;

Fx_RL     =    D_x_RL*sin(C_x_RL*atan(B_x_RL*K_x_RL - E_x_RL*(B_x_RL*K_x_RL-atan(B_x_RL*K_x_RL))))+S_Vx_RL;

Fx = [Fx_FR, Fx_FL, Fx_RR, Fx_RL]';
mux = [mux_FR, mux_FL, mux_RR, mux_RL]';
